simulink model "TIRE_forces_fl_fr"  (R2015a)
settings: Solver=ode45  StartTime=0.0  StopTime=10.0  RelTol=1e-3
settings Model: Creator=BML  LastModifiedBy=BML

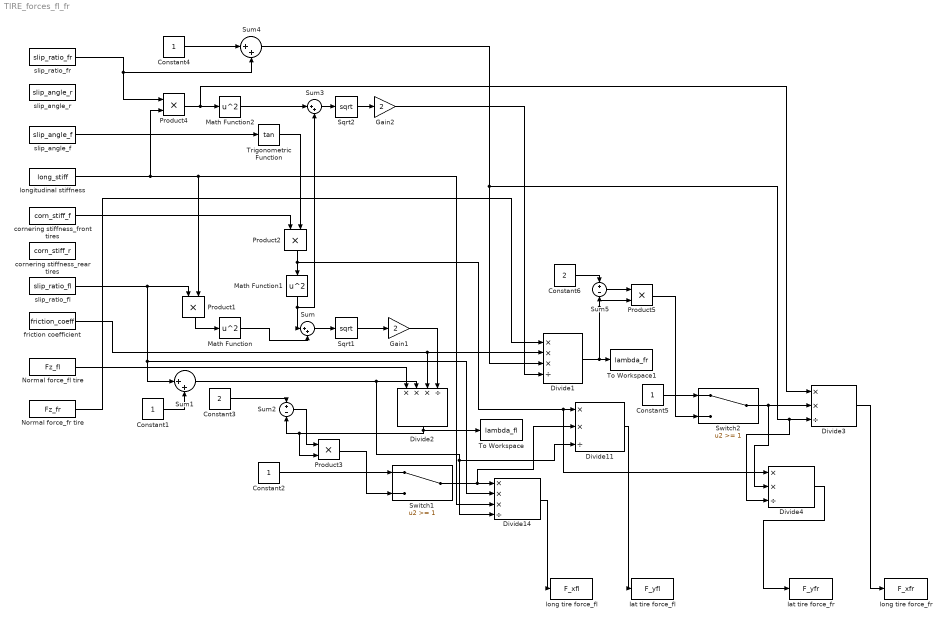
== system TIRE_forces_fl_fr ==
  Constant{1..2,4..5} (4 alike) : Constant
  Constant3 : Constant  Value=2
  Constant6 : Constant  Value=2
  Divide1 : Product  Inputs=***/
  Divide11 : Product  Inputs=**/
  Divide14 : Product  Inputs=***/
  Divide2 : Product  Inputs=***/
  Divide3 : Product  Inputs=**/
  Divide4 : Product  Inputs=**/
  Gain1 : Gain  Gain=2
  Gain2 : Gain  Gain=2
  Math Function : Math  Operator=square  SaturateOnIntegerOverflow=on
  Math Function1 : Math  Operator=square  SaturateOnIntegerOverflow=on
  Math Function2 : Math  Operator=square  SaturateOnIntegerOverflow=on
  Normal force_fl tire : FromWorkspace  VariableName=Fz_fl  SampleTime=0
  Normal force_fr tire : FromWorkspace  VariableName=Fz_fr  SampleTime=0
  Product{1..5} (5 alike) : Product
  Sqrt1 : Sqrt  SaturateOnIntegerOverflow=on
  Sqrt2 : Sqrt  SaturateOnIntegerOverflow=on
  Sum{,1,3..4} (4 alike) : Sum  Inputs=|++
  Sum2 : Sum  Inputs=+-
  Sum5 : Sum  Inputs=+-
  Switch1 : Switch  Threshold=1
  Switch2 : Switch  Threshold=1
  To Workspace : ToWorkspace  VariableName=lambda_fl  SaveFormat=Timeseries  SampleTime=-1
  To Workspace1 : ToWorkspace  VariableName=lambda_fr  SaveFormat=Timeseries  SampleTime=-1
  Trigonometric Function : Trigonometry  Operator=tan
  cornering stiffness_front tires : FromWorkspace  VariableName=corn_stiff_f  SampleTime=0
  cornering stiffness_rear tires : FromWorkspace  VariableName=corn_stiff_r  SampleTime=0
  friction coefficient : FromWorkspace  VariableName=friction_coeff  SampleTime=0
  lat tire force_fl : ToWorkspace  VariableName=F_yfl  SaveFormat=Timeseries  SampleTime=-1
  lat tire force_fr : ToWorkspace  VariableName=F_yfr  SaveFormat=Timeseries  SampleTime=-1
  long tire force_fl : ToWorkspace  VariableName=F_xfl  SaveFormat=Timeseries  SampleTime=-1
  long tire force_fr : ToWorkspace  VariableName=F_xfr  SaveFormat=Timeseries  SampleTime=-1
  longitudinal stiffness : FromWorkspace  VariableName=long_stiff  SampleTime=0
  slip_angle_f : FromWorkspace  VariableName=slip_angle_f  SampleTime=0
  slip_angle_r : FromWorkspace  VariableName=slip_angle_r  SampleTime=0
  slip_ratio_fl : FromWorkspace  VariableName=slip_ratio_fl  SampleTime=0
  slip_ratio_fr : FromWorkspace  VariableName=slip_ratio_fr  SampleTime=0
  wires:
  Product1/1 -> Math Function/1
  slip_angle_f/1 -> Trigonometric Function/1
  Trigonometric Function/1 -> Product2/2
  Math Function/1 -> Sum/2
  Sum/1 -> Sqrt1/1
  Sqrt1/1 -> Gain1/1
  Constant1/1 -> Sum1/2
  slip_ratio_fl/1 -> Divide14/2, Sum1/1, Product1/1
  Gain1/1 -> Divide2/4
  Normal force_fl tire/1 -> Divide2/1
  friction coefficient/1 -> Divide1/2, Divide2/3
  Constant2/1 -> Switch1/1
  Constant3/1 -> Sum2/1
  Sum2/1 -> Product3/1
  Divide2/1 -> Product3/2, Sum2/2, To Workspace/1
  Product3/1 -> Switch1/3
  Sum1/1 -> Divide11/3, Divide14/4, Divide2/2
  longitudinal stiffness/1 -> Product4/2, Product1/2, Divide14/3
  Divide14/1 -> long tire force_fl/1
  cornering stiffness_front tires/1 -> Product2/1
  Switch1/1 -> Divide11/2, Divide14/1
  Divide11/1 -> lat tire force_fl/1
  Normal force_fr tire/1 -> Divide1/1
  Math Function1/1 -> Sum3/2, Sum/1
  slip_ratio_fr/1 -> Sum4/2, Product4/1
  Math Function2/1 -> Sum3/1
  Sum3/1 -> Sqrt2/1
  Sqrt2/1 -> Gain2/1
  Gain2/1 -> Divide1/4
  Constant4/1 -> Sum4/1
  Product2/1 -> Divide4/1, Divide11/1, Math Function1/1
  Constant6/1 -> Sum5/1
  Divide1/1 -> Product5/2, Sum5/2, To Workspace1/1
  Sum5/1 -> Product5/1
  Product5/1 -> Switch2/3
  Constant5/1 -> Switch2/1
  Switch2/1 -> Divide4/2, Divide3/2
  Product4/1 -> Divide3/1, Math Function2/1
  Sum4/1 -> Divide4/3, Divide3/3, Divide1/3
  Divide3/1 -> long tire force_fr/1
  Divide4/1 -> lat tire force_fr/1
